simulink model "SVM"  (R2018b)
settings: Solver=VariableStepAuto  StartTime=0.0  StopTime=0.1  FixedStep=1/100000000  RelTol=1e-3
PostLoadFcn:
  | , if any(exist('dsrtsu_mdlpostloadfcn', 'file') ~= 0), dsrtsu_mdlpostloadfcn('Execute', bdroot); end,
values from neighbouring files (symbols this model uses):
  omega = 75    [param.m]
  Vo = 200    [param.m]
libraries: xbsIndex_r4 x2079, xrbsSSR_Library x20, xrbsMath_r4 x11, rtiproclib x6, rtifpgainterfacelib x1, powerlib_meascontrol x1
(part 5 of 23)

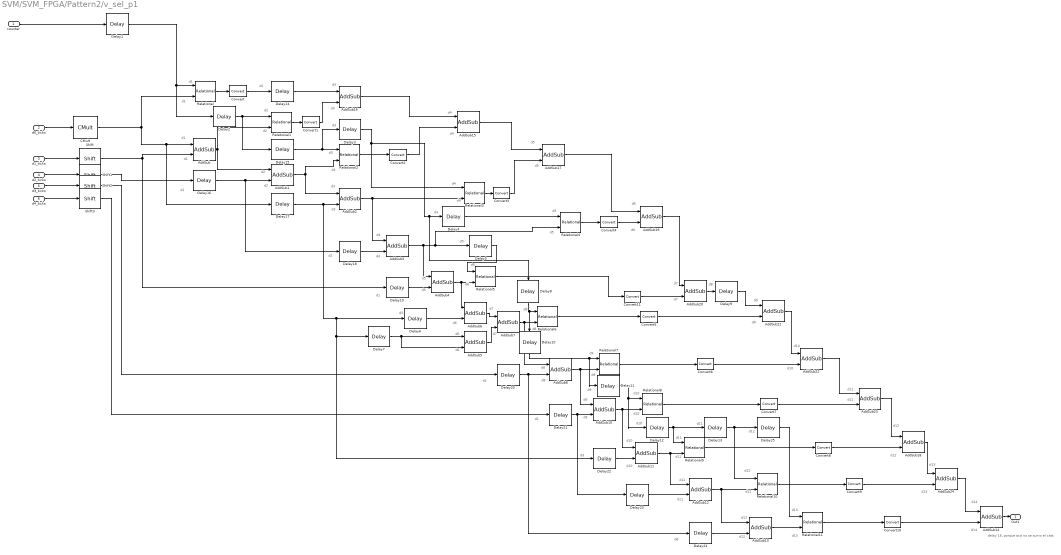
== system SVM/SVM_FPGA/Pattern2/v_sel_p1 ==
  note: d14
  note: d13
  note: d14
  note: d13
  note: d12
  note: d13
  note: d12
  note: d12
  note: d11
  note: d12
  note: d11
  note: d12
  note: d11
  note: d13
  note: d12
  note: d11
  note: d10
  note: d11
  note: d10
  note: d10
  note: d3
  note: d9
  note: d1
  note: d12
  note: d11
  note: d9
  note: d10
  note: d10
  note: d9
  note: d8
  note: d11
  note: d10
  note: d9
  note: d9
  note: d8
  note: d1
  note: d8
  note: d10
  note: d9
  note: d8
  note: d9
  note: d8
  note: d6
  note: d5
  note: d4
  note: d8
  note: d7
  note: d7
  note: d6
  note: d6
  note: d1
  note: d2
  note: d3
  note: d6
  note: d7
  note: d7
  note: d5
  note: d6
  note: d6
  note: d5
  note: d5
  note: d5
  note: d4
  note: d4
  note: d6
  note: d5
  note: d3
  note: d4
  note: d4
  note: d3
  note: d3
  note: d4
  note: d3
  note: d2
  note: d2
  note: d3
  note: d3
  note: d2
  note: d2
  note: d1
  note: d1
  note: d1
  note: d1
  note: d5
  note: d4
  note: d3
  note: d2
  note: d1
  note: delay 16, porque acá no se sumo el cast
  counter : Inport
  d0_ticks : Inport  Port=2
  d1_ticks : Inport  Port=3
  d2_ticks : Inport  Port=4
  d3_ticks : Inport  Port=5
  d4_ticks : Inport  Port=6
  AddSub{,1..8,10..13} (13 alike) : xbsIndex_r4/AddSub  mode=Addition  use_carryin=off  use_carryout=off  en=off  latency=1  precision=Full  arith_type=Unsigned  n_bits=16  bin_pt=14  quantization=Truncate  overflow=Wrap  use_behavioral_HDL=off  hw_selection=Fabric  pipelined=off  dbl_ovrd=off  block_type=addsub
  AddSub{14,18,22..24} (5 alike) : xbsIndex_r4/AddSub  mode=Addition  use_carryin=off  use_carryout=off  en=off  latency=1  precision=User Defined  arith_type=Unsigned  n_bits=4  bin_pt=0  quantization=Truncate  overflow=Wrap  use_behavioral_HDL=off  hw_selection=Fabric  pipelined=off  dbl_ovrd=off  block_type=addsub
  AddSub15 : xbsIndex_r4/AddSub  mode=Addition  use_carryin=off  use_carryout=off  en=off  latency=1  precision=User Defined  arith_type=Unsigned  n_bits=2  bin_pt=0  quantization=Truncate  overflow=Wrap  use_behavioral_HDL=off  hw_selection=Fabric  pipelined=off  dbl_ovrd=off  block_type=addsub
  AddSub16 : xbsIndex_r4/AddSub  mode=Addition  use_carryin=off  use_carryout=off  en=off  latency=1  precision=User Defined  arith_type=Unsigned  n_bits=2  bin_pt=0  quantization=Truncate  overflow=Wrap  use_behavioral_HDL=off  hw_selection=Fabric  pipelined=off  dbl_ovrd=off  block_type=addsub
  AddSub{17,19..21} (4 alike) : xbsIndex_r4/AddSub  mode=Addition  use_carryin=off  use_carryout=off  en=off  latency=1  precision=User Defined  arith_type=Unsigned  n_bits=3  bin_pt=0  quantization=Truncate  overflow=Wrap  use_behavioral_HDL=off  hw_selection=Fabric  pipelined=off  dbl_ovrd=off  block_type=addsub
  CMult : xbsIndex_r4/CMult  const=1/6  gui_display_data_type=Fixed-point  const_n_bits=16  const_bin_pt=16  float_type=Single  exp_bits=8  fraction_bits=24  en=off  latency=1  precision=Full  arith_type="Signed  (2's comp)"  n_bits=16  bin_pt=14  quantization=Truncate  overflow=Wrap  use_behavioral_HDL=off  mem_type=Distributed RAM  pipeline=off  dbl_ovrd=off  block_type=cmult
  Convert{,1..11} (12 alike) : xbsIndex_r4/Convert  gui_display_data_type=Fixed-point  arith_type="Signed  (2's comp)"  n_bits=1  bin_pt=0  float_type=Single  exp_bits=8  fraction_bits=24  quantization=Truncate  overflow=Wrap  en=off  latency=1  pipeline=off  dbl_ovrd=off  block_type=convert
  Delay{1..5,9..16,25} (14 alike) : xbsIndex_r4/Delay  rst=off  infoeditControl=Selection of Reset will increase slice count due to use of real FFs and instead of SRLs  en=off  latency=1  reg_retiming=off  dbl_ovrd=off  block_type=delay
  Delay17 : xbsIndex_r4/Delay  rst=off  infoeditControl=Selection of Reset will increase slice count due to use of real FFs and instead of SRLs  en=off  latency=2  reg_retiming=off  dbl_ovrd=off  block_type=delay
  Delay18 : xbsIndex_r4/Delay  rst=off  infoeditControl=Selection of Reset will increase slice count due to use of real FFs and instead of SRLs  en=off  latency=2  reg_retiming=off  dbl_ovrd=off  block_type=delay
  Delay19 : xbsIndex_r4/Delay  rst=off  infoeditControl=Selection of Reset will increase slice count due to use of real FFs and instead of SRLs  en=off  latency=4  reg_retiming=off  dbl_ovrd=off  block_type=delay
  Delay20 : xbsIndex_r4/Delay  rst=off  infoeditControl=Selection of Reset will increase slice count due to use of real FFs and instead of SRLs  en=off  latency=7  reg_retiming=off  dbl_ovrd=off  block_type=delay
  Delay21 : xbsIndex_r4/Delay  rst=off  infoeditControl=Selection of Reset will increase slice count due to use of real FFs and instead of SRLs  en=off  latency=8  reg_retiming=off  dbl_ovrd=off  block_type=delay
  Delay22 : xbsIndex_r4/Delay  rst=off  infoeditControl=Selection of Reset will increase slice count due to use of real FFs and instead of SRLs  en=off  latency=7  reg_retiming=off  dbl_ovrd=off  block_type=delay
  Delay23 : xbsIndex_r4/Delay  rst=off  infoeditControl=Selection of Reset will increase slice count due to use of real FFs and instead of SRLs  en=off  latency=2  reg_retiming=off  dbl_ovrd=off  block_type=delay
  Delay24 : xbsIndex_r4/Delay  rst=off  infoeditControl=Selection of Reset will increase slice count due to use of real FFs and instead of SRLs  en=off  latency=4  reg_retiming=off  dbl_ovrd=off  block_type=delay
  Delay6 : xbsIndex_r4/Delay  rst=off  infoeditControl=Selection of Reset will increase slice count due to use of real FFs and instead of SRLs  en=off  latency=3  reg_retiming=off  dbl_ovrd=off  block_type=delay
  Delay7 : xbsIndex_r4/Delay  rst=off  infoeditControl=Selection of Reset will increase slice count due to use of real FFs and instead of SRLs  en=off  latency=3  reg_retiming=off  dbl_ovrd=off  block_type=delay
  Delay8 : xbsIndex_r4/Delay  rst=off  infoeditControl=Selection of Reset will increase slice count due to use of real FFs and instead of SRLs  en=off  latency=4  reg_retiming=off  dbl_ovrd=off  block_type=delay
  Relational{,1..11} (12 alike) : xbsIndex_r4/Relational  mode=a>b  op_type=Bool  en=off  latency=1  dbl_ovrd=off  block_type=relational
  Shift{,1..3} (4 alike) : xbsIndex_r4/Shift  shift_dir=Right  shift_bits=1  en=off  latency=1  precision=Full  arith_type="Signed  (2's comp)"  n_bits=16  bin_pt=14  quantization=Truncate  overflow=Wrap  dbl_ovrd=off  block_type=shift
  Out1 : Outport
  wires:
  AddSub15/1 -> AddSub17/1
  AddSub16/1 -> AddSub15/1
  AddSub24/1 -> AddSub14/1
  Shift1/1 -> Delay16/1
  Delay17/1 -> AddSub2/2, Delay22/1, Delay7/1, Delay6/1
  AddSub20/1 -> Delay9/1
  AddSub11/1 -> AddSub12/1, Relational9/2
  AddSub6/1 -> AddSub7/1
  Relational4/1 -> Convert4/1
  Delay19/1 -> AddSub4/2
  counter/1 -> Delay1/1
  AddSub18/1 -> AddSub24/1
  CMult/1 -> Delay17/1, AddSub/1, Relational/2
  Shift/1 -> Delay19/1, AddSub/2
  Delay20/1 -> Delay24/1, AddSub8/2
  Delay22/1 -> AddSub11/2
  AddSub5/1 -> AddSub7/2
  Delay16/1 -> Delay18/1, AddSub1/2
  Relational1/1 -> Convert1/1
  AddSub12/1 -> AddSub13/1, Relational10/2
  Relational8/1 -> Convert7/1
  AddSub23/1 -> AddSub18/1
  Delay23/1 -> AddSub12/2
  Relational5/1 -> Convert11/1
  AddSub4/1 -> AddSub6/1, Relational5/2
  AddSub/1 -> AddSub1/1, Relational1/2
  AddSub8/1 -> AddSub10/1, Relational7/2
  Delay15/1 -> Delay3/1, Relational2/1
  AddSub7/1 -> Relational6/2, AddSub8/1
  Relational2/1 -> Convert2/1
  Delay21/1 -> Delay23/1, AddSub10/2
  d3_ticks/1 -> Shift2/1
  Relational6/1 -> Convert5/1
  Relational10/1 -> Convert9/1
  AddSub19/1 -> AddSub20/1
  Delay18/1 -> AddSub3/2
  AddSub17/1 -> AddSub19/1
  Relational/1 -> Convert/1
  AddSub1/1 -> AddSub2/1, Relational2/2
  AddSub22/1 -> AddSub23/1
  AddSub3/1 -> AddSub4/1, Relational4/2, Delay5/1
  AddSub10/1 -> AddSub11/1, Relational8/2
  d1_ticks/1 -> Shift/1
  AddSub13/1 -> Relational11/2
  Delay24/1 -> AddSub13/2
  d0_ticks/1 -> CMult/1
  Shift2/1 -> Delay20/1
  Relational3/1 -> Convert3/1
  Relational11/1 -> Convert10/1
  AddSub2/1 -> AddSub3/1, Relational3/2
  AddSub21/1 -> AddSub22/1
  Shift3/1 -> Delay21/1
  Relational7/1 -> Convert6/1
  Relational9/1 -> Convert8/1
  AddSub14/1 -> Out1/1
  d4_ticks/1 -> Shift3/1
  d2_ticks/1 -> Shift1/1
  Delay1/1 -> Delay2/1, Relational/1
  Delay2/1 -> Relational1/1, Delay15/1
  Delay3/1 -> Relational3/1, Delay8/1, Delay4/1
  Delay4/1 -> Relational4/1
  Delay5/1 -> Relational5/1
  Delay6/1 -> AddSub6/2
  Delay7/1 -> AddSub5/2, AddSub5/1
  Delay8/1 -> Delay10/1, Relational6/1
  Delay9/1 -> AddSub21/1
  Delay10/1 -> Delay11/1, Relational7/1
  Delay11/1 -> Delay12/1, Relational8/1
  Delay12/1 -> Relational9/1, Delay13/1
  Delay13/1 -> Relational10/1, Delay25/1
  Delay25/1 -> Relational11/1
  Delay14/1 -> AddSub16/1
  Convert1/1 -> AddSub16/2
  Convert2/1 -> AddSub15/2
  Convert3/1 -> AddSub17/2
  Convert4/1 -> AddSub19/2
  Convert5/1 -> AddSub21/2
  Convert6/1 -> AddSub22/2
  Convert7/1 -> AddSub23/2
  Convert8/1 -> AddSub18/2
  Convert9/1 -> AddSub24/2
  Convert10/1 -> AddSub14/2
  Convert11/1 -> AddSub20/2
  Convert/1 -> Delay14/1

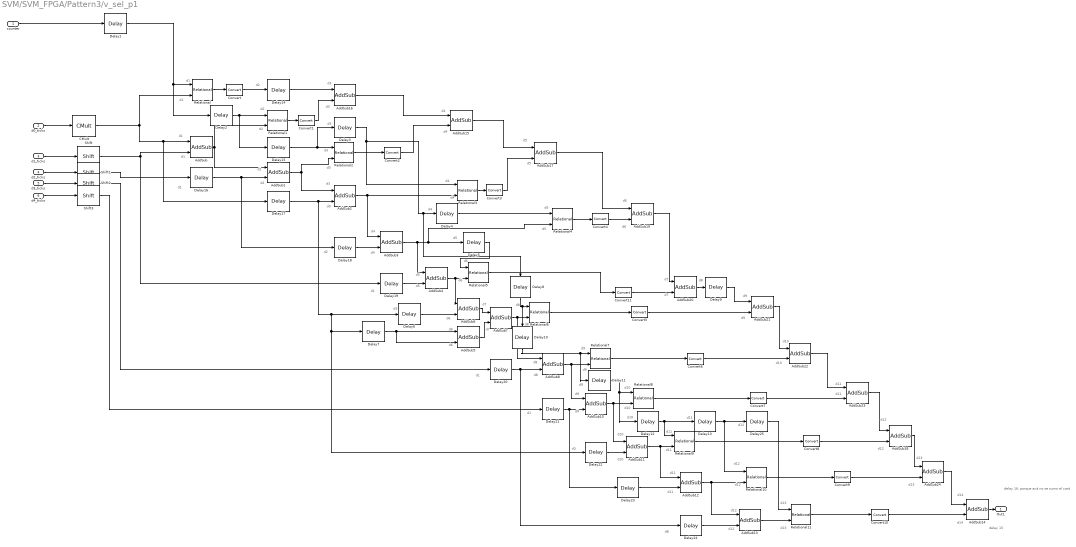
== system SVM/SVM_FPGA/Pattern3/v_sel_p1 ==
  note: delay 15
  note: d1
  note: d2
  note: d3
  note: d4
  note: d5
  note: d1
  note: d1
  note: d1
  note: d1
  note: d2
  note: d2
  note: d3
  note: d3
  note: d2
  note: d2
  note: d3
  note: d4
  note: d3
  note: d3
  note: d4
  note: d4
  note: d3
  note: d5
  note: d6
  note: d4
  note: d4
  note: d5
  note: d5
  note: d5
  note: d6
  note: d6
  note: d5
  note: d7
  note: d7
  note: d6
  note: d3
  note: d2
  note: d1
  note: d6
  note: d6
  note: d7
  note: d7
  note: d8
  note: d4
  note: d5
  note: d6
  note: d8
  note: d9
  note: d8
  note: d9
  note: d10
  note: d8
  note: d1
  note: d8
  note: d9
  note: d9
  note: d10
  note: d11
  note: d8
  note: d9
  note: d10
  note: d10
  note: d9
  note: d11
  note: d12
  note: d1
  note: d9
  note: d3
  note: d10
  note: d10
  note: d11
  note: d10
  note: d11
  note: d12
  note: d13
  note: d11
  note: d12
  note: d11
  note: d12
  note: d11
  note: d12
  note: d12
  note: d13
  note: d12
  note: d13
  note: d14
  note: d13
  note: d14
  note: delay 16, porque acá no se sumo el cast
  counter : Inport
  d0_ticks : Inport  Port=2
  d1_ticks : Inport  Port=3
  d2_ticks : Inport  Port=4
  d3_ticks : Inport  Port=5
  d4_ticks : Inport  Port=6
  AddSub{,1..8,10..13} (13 alike) : xbsIndex_r4/AddSub  mode=Addition  use_carryin=off  use_carryout=off  en=off  latency=1  precision=Full  arith_type=Unsigned  n_bits=16  bin_pt=14  quantization=Truncate  overflow=Wrap  use_behavioral_HDL=off  hw_selection=Fabric  pipelined=off  dbl_ovrd=off  block_type=addsub
  AddSub{14,18,22..24} (5 alike) : xbsIndex_r4/AddSub  mode=Addition  use_carryin=off  use_carryout=off  en=off  latency=1  precision=User Defined  arith_type=Unsigned  n_bits=4  bin_pt=0  quantization=Truncate  overflow=Wrap  use_behavioral_HDL=off  hw_selection=Fabric  pipelined=off  dbl_ovrd=off  block_type=addsub
  AddSub15 : xbsIndex_r4/AddSub  mode=Addition  use_carryin=off  use_carryout=off  en=off  latency=1  precision=User Defined  arith_type=Unsigned  n_bits=2  bin_pt=0  quantization=Truncate  overflow=Wrap  use_behavioral_HDL=off  hw_selection=Fabric  pipelined=off  dbl_ovrd=off  block_type=addsub
  AddSub16 : xbsIndex_r4/AddSub  mode=Addition  use_carryin=off  use_carryout=off  en=off  latency=1  precision=User Defined  arith_type=Unsigned  n_bits=2  bin_pt=0  quantization=Truncate  overflow=Wrap  use_behavioral_HDL=off  hw_selection=Fabric  pipelined=off  dbl_ovrd=off  block_type=addsub
  AddSub{17,19..21} (4 alike) : xbsIndex_r4/AddSub  mode=Addition  use_carryin=off  use_carryout=off  en=off  latency=1  precision=User Defined  arith_type=Unsigned  n_bits=3  bin_pt=0  quantization=Truncate  overflow=Wrap  use_behavioral_HDL=off  hw_selection=Fabric  pipelined=off  dbl_ovrd=off  block_type=addsub
  CMult : xbsIndex_r4/CMult  const=1/6  gui_display_data_type=Fixed-point  const_n_bits=16  const_bin_pt=16  float_type=Single  exp_bits=8  fraction_bits=24  en=off  latency=1  precision=Full  arith_type="Signed  (2's comp)"  n_bits=16  bin_pt=14  quantization=Truncate  overflow=Wrap  use_behavioral_HDL=off  mem_type=Distributed RAM  pipeline=off  dbl_ovrd=off  block_type=cmult
  Convert{,1..11} (12 alike) : xbsIndex_r4/Convert  gui_display_data_type=Fixed-point  arith_type="Signed  (2's comp)"  n_bits=1  bin_pt=0  float_type=Single  exp_bits=8  fraction_bits=24  quantization=Truncate  overflow=Wrap  en=off  latency=1  pipeline=off  dbl_ovrd=off  block_type=convert
  Delay{1..5,9..16,25} (14 alike) : xbsIndex_r4/Delay  rst=off  infoeditControl=Selection of Reset will increase slice count due to use of real FFs and instead of SRLs  en=off  latency=1  reg_retiming=off  dbl_ovrd=off  block_type=delay
  Delay17 : xbsIndex_r4/Delay  rst=off  infoeditControl=Selection of Reset will increase slice count due to use of real FFs and instead of SRLs  en=off  latency=2  reg_retiming=off  dbl_ovrd=off  block_type=delay
  Delay18 : xbsIndex_r4/Delay  rst=off  infoeditControl=Selection of Reset will increase slice count due to use of real FFs and instead of SRLs  en=off  latency=2  reg_retiming=off  dbl_ovrd=off  block_type=delay
  Delay19 : xbsIndex_r4/Delay  rst=off  infoeditControl=Selection of Reset will increase slice count due to use of real FFs and instead of SRLs  en=off  latency=4  reg_retiming=off  dbl_ovrd=off  block_type=delay
  Delay20 : xbsIndex_r4/Delay  rst=off  infoeditControl=Selection of Reset will increase slice count due to use of real FFs and instead of SRLs  en=off  latency=7  reg_retiming=off  dbl_ovrd=off  block_type=delay
  Delay21 : xbsIndex_r4/Delay  rst=off  infoeditControl=Selection of Reset will increase slice count due to use of real FFs and instead of SRLs  en=off  latency=8  reg_retiming=off  dbl_ovrd=off  block_type=delay
  Delay22 : xbsIndex_r4/Delay  rst=off  infoeditControl=Selection of Reset will increase slice count due to use of real FFs and instead of SRLs  en=off  latency=7  reg_retiming=off  dbl_ovrd=off  block_type=delay
  Delay23 : xbsIndex_r4/Delay  rst=off  infoeditControl=Selection of Reset will increase slice count due to use of real FFs and instead of SRLs  en=off  latency=2  reg_retiming=off  dbl_ovrd=off  block_type=delay
  Delay24 : xbsIndex_r4/Delay  rst=off  infoeditControl=Selection of Reset will increase slice count due to use of real FFs and instead of SRLs  en=off  latency=4  reg_retiming=off  dbl_ovrd=off  block_type=delay
  Delay6 : xbsIndex_r4/Delay  rst=off  infoeditControl=Selection of Reset will increase slice count due to use of real FFs and instead of SRLs  en=off  latency=3  reg_retiming=off  dbl_ovrd=off  block_type=delay
  Delay7 : xbsIndex_r4/Delay  rst=off  infoeditControl=Selection of Reset will increase slice count due to use of real FFs and instead of SRLs  en=off  latency=3  reg_retiming=off  dbl_ovrd=off  block_type=delay
  Delay8 : xbsIndex_r4/Delay  rst=off  infoeditControl=Selection of Reset will increase slice count due to use of real FFs and instead of SRLs  en=off  latency=4  reg_retiming=off  dbl_ovrd=off  block_type=delay
  Relational{,1..11} (12 alike) : xbsIndex_r4/Relational  mode=a>b  op_type=Bool  en=off  latency=1  dbl_ovrd=off  block_type=relational
  Shift{,1..3} (4 alike) : xbsIndex_r4/Shift  shift_dir=Right  shift_bits=1  en=off  latency=1  precision=Full  arith_type="Signed  (2's comp)"  n_bits=16  bin_pt=14  quantization=Truncate  overflow=Wrap  dbl_ovrd=off  block_type=shift
  Out1 : Outport
  wires:
  Convert/1 -> Delay14/1
  Convert11/1 -> AddSub20/2
  Convert10/1 -> AddSub14/2
  Convert9/1 -> AddSub24/2
  Convert8/1 -> AddSub18/2
  Convert7/1 -> AddSub23/2
  Convert6/1 -> AddSub22/2
  Convert5/1 -> AddSub21/2
  Convert4/1 -> AddSub19/2
  Convert3/1 -> AddSub17/2
  Convert2/1 -> AddSub15/2
  Convert1/1 -> AddSub16/2
  Delay14/1 -> AddSub16/1
  Delay25/1 -> Relational11/1
  Delay13/1 -> Delay25/1, Relational10/1
  Delay12/1 -> Delay13/1, Relational9/1
  Delay11/1 -> Relational8/1, Delay12/1
  Delay10/1 -> Relational7/1, Delay11/1
  Delay9/1 -> AddSub21/1
  Delay8/1 -> Relational6/1, Delay10/1
  Delay7/1 -> AddSub5/1, AddSub5/2
  Delay6/1 -> AddSub6/2
  Delay5/1 -> Relational5/1
  Delay4/1 -> Relational4/1
  Delay3/1 -> Delay4/1, Delay8/1, Relational3/1
  Delay2/1 -> Delay15/1, Relational1/1
  Delay1/1 -> Relational/1, Delay2/1
  d2_ticks/1 -> Shift1/1
  d4_ticks/1 -> Shift3/1
  AddSub14/1 -> Out1/1
  Relational9/1 -> Convert8/1
  Relational7/1 -> Convert6/1
  Shift3/1 -> Delay21/1
  AddSub21/1 -> AddSub22/1
  AddSub2/1 -> Relational3/2, AddSub3/1
  Relational11/1 -> Convert10/1
  Relational3/1 -> Convert3/1
  Shift2/1 -> Delay20/1
  d0_ticks/1 -> CMult/1
  Delay24/1 -> AddSub13/2
  AddSub13/1 -> Relational11/2
  d1_ticks/1 -> Shift/1
  AddSub10/1 -> Relational8/2, AddSub11/1
  AddSub3/1 -> Delay5/1, Relational4/2, AddSub4/1
  AddSub22/1 -> AddSub23/1
  AddSub1/1 -> Relational2/2, AddSub2/1
  Relational/1 -> Convert/1
  AddSub17/1 -> AddSub19/1
  Delay18/1 -> AddSub3/2
  AddSub19/1 -> AddSub20/1
  Relational10/1 -> Convert9/1
  Relational6/1 -> Convert5/1
  d3_ticks/1 -> Shift2/1
  Delay21/1 -> AddSub10/2, Delay23/1
  Relational2/1 -> Convert2/1
  AddSub7/1 -> AddSub8/1, Relational6/2
  Delay15/1 -> Relational2/1, Delay3/1
  AddSub8/1 -> Relational7/2, AddSub10/1
  AddSub/1 -> Relational1/2, AddSub1/1
  AddSub4/1 -> Relational5/2, AddSub6/1
  Relational5/1 -> Convert11/1
  Delay23/1 -> AddSub12/2
  AddSub23/1 -> AddSub18/1
  Relational8/1 -> Convert7/1
  AddSub12/1 -> Relational10/2, AddSub13/1
  Relational1/1 -> Convert1/1
  Delay16/1 -> AddSub1/2, Delay18/1
  AddSub5/1 -> AddSub7/2
  Delay22/1 -> AddSub11/2
  Delay20/1 -> AddSub8/2, Delay24/1
  Shift/1 -> AddSub/2, Delay19/1
  CMult/1 -> Relational/2, AddSub/1, Delay17/1
  AddSub18/1 -> AddSub24/1
  counter/1 -> Delay1/1
  Delay19/1 -> AddSub4/2
  Relational4/1 -> Convert4/1
  AddSub6/1 -> AddSub7/1
  AddSub11/1 -> Relational9/2, AddSub12/1
  AddSub20/1 -> Delay9/1
  Delay17/1 -> Delay6/1, Delay7/1, Delay22/1, AddSub2/2
  Shift1/1 -> Delay16/1
  AddSub24/1 -> AddSub14/1
  AddSub16/1 -> AddSub15/1
  AddSub15/1 -> AddSub17/1

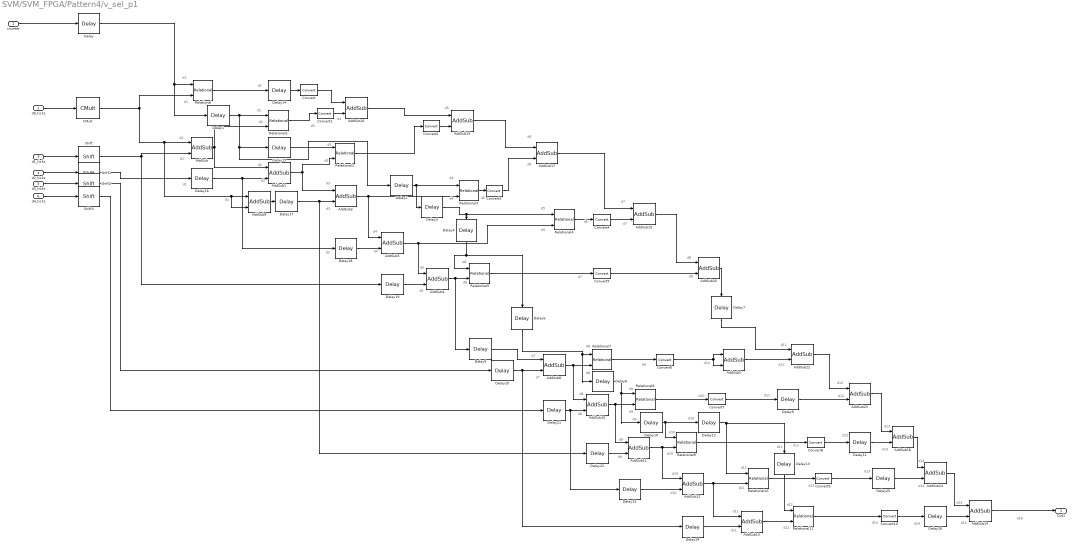
== system SVM/SVM_FPGA/Pattern4/v_sel_p1 ==
  note: d16
  note: d15
  note: d14
  note: d15
  note: d14
  note: d13
  note: d12
  note: d13
  note: d12
  note: d11
  note: d12
  note: d11
  note: d11
  note: d11
  note: d10
  note: d9
  note: d11
  note: d10
  note: d10
  note: d14
  note: d12
  note: d13
  note: d11
  note: d10
  note: d10
  note: d9
  note: d9
  note: d13
  note: d12
  note: d11
  note: d12
  note: d10
  note: d9
  note: d9
  note: d8
  note: d8
  note: d8
  note: d8
  note: d9
  note: d10
  note: d11
  note: d7
  note: d7
  note: d11
  note: d8
  note: d7
  note: d6
  note: d6
  note: d5
  note: d5
  note: d8
  note: d7
  note: d6
  note: d5
  note: d5
  note: d4
  note: d4
  note: d6
  note: d5
  note: d4
  note: d3
  note: d3
  note: d4
  note: d3
  note: d2
  note: d2
  note: d3
  note: d2
  note: d2
  note: d3
  note: d4
  note: d2
  note: d1
  note: d1
  note: d1
  note: d1
  note: d2
  note: d1
  note: d1
  note: d7
  note: d6
  note: d5
  counter : Inport
  d0_ticks : Inport  Port=2
  d1_ticks : Inport  Port=3
  d2_ticks : Inport  Port=4
  d3_ticks : Inport  Port=5
  d4_ticks : Inport  Port=6
  AddSub{,1..5,8..13,16} (13 alike) : xbsIndex_r4/AddSub  mode=Addition  use_carryin=off  use_carryout=off  en=off  latency=1  precision=Full  arith_type=Unsigned  n_bits=16  bin_pt=14  quantization=Truncate  overflow=Wrap  use_behavioral_HDL=off  hw_selection=Fabric  pipelined=off  dbl_ovrd=off  block_type=addsub
  AddSub{14,18,23..24} (4 alike) : xbsIndex_r4/AddSub  mode=Addition  use_carryin=off  use_carryout=off  en=off  latency=1  precision=User Defined  arith_type=Unsigned  n_bits=4  bin_pt=0  quantization=Truncate  overflow=Wrap  use_behavioral_HDL=off  hw_selection=Fabric  pipelined=off  dbl_ovrd=off  block_type=addsub
  AddSub15 : xbsIndex_r4/AddSub  mode=Addition  use_carryin=off  use_carryout=off  en=off  latency=1  precision=User Defined  arith_type=Unsigned  n_bits=2  bin_pt=0  quantization=Truncate  overflow=Wrap  use_behavioral_HDL=off  hw_selection=Fabric  pipelined=off  dbl_ovrd=off  block_type=addsub
  AddSub17 : xbsIndex_r4/AddSub  mode=Addition  use_carryin=off  use_carryout=off  en=off  latency=1  precision=User Defined  arith_type=Unsigned  n_bits=3  bin_pt=0  quantization=Truncate  overflow=Wrap  use_behavioral_HDL=off  hw_selection=Fabric  pipelined=off  dbl_ovrd=off  block_type=addsub
  AddSub19 : xbsIndex_r4/AddSub  mode=Addition  use_carryin=off  use_carryout=off  en=off  latency=1  precision=User Defined  arith_type=Unsigned  n_bits=3  bin_pt=0  quantization=Truncate  overflow=Wrap  use_behavioral_HDL=off  hw_selection=Fabric  pipelined=off  dbl_ovrd=off  block_type=addsub
  AddSub20 : xbsIndex_r4/AddSub  mode=Addition  use_carryin=off  use_carryout=off  en=off  latency=1  precision=User Defined  arith_type=Unsigned  n_bits=5  bin_pt=0  quantization=Truncate  overflow=Wrap  use_behavioral_HDL=off  hw_selection=Fabric  pipelined=off  dbl_ovrd=off  block_type=addsub
  AddSub22 : xbsIndex_r4/AddSub  mode=Addition  use_carryin=off  use_carryout=off  en=off  latency=1  precision=User Defined  arith_type=Unsigned  n_bits=3  bin_pt=0  quantization=Truncate  overflow=Wrap  use_behavioral_HDL=off  hw_selection=Fabric  pipelined=off  dbl_ovrd=off  block_type=addsub
  CMult : xbsIndex_r4/CMult  const=1/6  gui_display_data_type=Fixed-point  const_n_bits=16  const_bin_pt=16  float_type=Single  exp_bits=8  fraction_bits=24  en=off  latency=1  precision=Full  arith_type="Signed  (2's comp)"  n_bits=16  bin_pt=14  quantization=Truncate  overflow=Wrap  use_behavioral_HDL=off  mem_type=Distributed RAM  pipeline=off  dbl_ovrd=off  block_type=cmult
  Convert{,1..10} (11 alike) : xbsIndex_r4/Convert  gui_display_data_type=Fixed-point  arith_type="Signed  (2's comp)"  n_bits=1  bin_pt=0  float_type=Single  exp_bits=8  fraction_bits=24  quantization=Truncate  overflow=Wrap  en=off  latency=1  pipeline=off  dbl_ovrd=off  block_type=convert
  Delay{,1,3..5,8..17,25..26} (17 alike) : xbsIndex_r4/Delay  rst=off  infoeditControl=Selection of Reset will increase slice count due to use of real FFs and instead of SRLs  en=off  latency=1  reg_retiming=off  dbl_ovrd=off  block_type=delay
  Delay{2,6..7,18,23} (5 alike) : xbsIndex_r4/Delay  rst=off  infoeditControl=Selection of Reset will increase slice count due to use of real FFs and instead of SRLs  en=off  latency=2  reg_retiming=off  dbl_ovrd=off  block_type=delay
  Delay19 : xbsIndex_r4/Delay  rst=off  infoeditControl=Selection of Reset will increase slice count due to use of real FFs and instead of SRLs  en=off  latency=4  reg_retiming=off  dbl_ovrd=off  block_type=delay
  Delay20 : xbsIndex_r4/Delay  rst=off  infoeditControl=Selection of Reset will increase slice count due to use of real FFs and instead of SRLs  en=off  latency=6  reg_retiming=off  dbl_ovrd=off  block_type=delay
  Delay21 : xbsIndex_r4/Delay  rst=off  infoeditControl=Selection of Reset will increase slice count due to use of real FFs and instead of SRLs  en=off  latency=7  reg_retiming=off  dbl_ovrd=off  block_type=delay
  Delay22 : xbsIndex_r4/Delay  rst=off  infoeditControl=Selection of Reset will increase slice count due to use of real FFs and instead of SRLs  en=off  latency=6  reg_retiming=off  dbl_ovrd=off  block_type=delay
  Delay24 : xbsIndex_r4/Delay  rst=off  infoeditControl=Selection of Reset will increase slice count due to use of real FFs and instead of SRLs  en=off  latency=4  reg_retiming=off  dbl_ovrd=off  block_type=delay
  Relational{,1..5,7..11} (11 alike) : xbsIndex_r4/Relational  mode=a>b  op_type=Bool  en=off  latency=1  dbl_ovrd=off  block_type=relational
  Shift{,1..3} (4 alike) : xbsIndex_r4/Shift  shift_dir=Right  shift_bits=1  en=off  latency=1  precision=Full  arith_type="Signed  (2's comp)"  n_bits=16  bin_pt=14  quantization=Truncate  overflow=Wrap  dbl_ovrd=off  block_type=shift
  Out1 : Outport
  wires:
  AddSub15/1 -> AddSub17/1
  AddSub24/1 -> AddSub14/1
  Shift1/1 -> Delay16/1
  Delay17/1 -> AddSub2/2, Delay22/1
  AddSub11/1 -> AddSub12/1, Relational9/2
  Relational4/1 -> Convert4/1
  Delay19/1 -> AddSub4/2
  counter/1 -> Delay/1
  AddSub18/1 -> AddSub24/1
  CMult/1 -> Relational/2, AddSub9/2, AddSub9/1, AddSub/1
  Shift/1 -> Delay19/1, AddSub/2
  Delay20/1 -> Delay24/1, AddSub8/2
  Delay22/1 -> AddSub11/2
  Delay16/1 -> Delay18/1, AddSub1/2
  Relational1/1 -> Convert1/1
  AddSub12/1 -> AddSub13/1, Relational10/2
  Relational8/1 -> Convert7/1
  AddSub23/1 -> AddSub18/1
  Delay23/1 -> AddSub12/2
  Relational5/1 -> Convert5/1
  AddSub4/1 -> Delay5/1, Relational5/2
  AddSub/1 -> AddSub1/1, Relational1/2
  AddSub8/1 -> AddSub10/1, Relational7/2
  Delay15/1 -> Relational2/1
  Relational2/1 -> Convert2/1
  Delay14/1 -> Convert/1
  Delay21/1 -> Delay23/1, AddSub10/2
  d3_ticks/1 -> Shift2/1
  Relational10/1 -> Convert9/1
  AddSub19/1 -> AddSub20/1
  Delay18/1 -> AddSub3/2
  AddSub17/1 -> AddSub19/1
  Relational/1 -> Delay14/1
  AddSub1/1 -> AddSub2/1, Relational2/2
  AddSub22/1 -> AddSub23/1
  AddSub3/1 -> AddSub4/1, Relational4/2
  AddSub10/1 -> AddSub11/1, Relational8/2
  d1_ticks/1 -> Shift/1
  AddSub13/1 -> Relational11/2
  Delay24/1 -> AddSub13/2
  Shift2/1 -> Delay20/1
  Relational3/1 -> Convert3/1
  Relational11/1 -> Convert10/1
  AddSub2/1 -> AddSub3/1, Relational3/2
  AddSub20/1 -> Delay7/1
  Shift3/1 -> Delay21/1
  Relational7/1 -> Convert6/1
  Relational9/1 -> Convert8/1
  AddSub14/1 -> Out1/1
  d4_ticks/1 -> Shift3/1
  d2_ticks/1 -> Shift1/1
  AddSub9/1 -> Delay17/1
  AddSub5/1 -> AddSub22/2
  d0_ticks/1 -> CMult/1
  Convert/1 -> AddSub16/1
  Convert1/1 -> AddSub16/2
  AddSub16/1 -> AddSub15/1
  Convert2/1 -> AddSub15/2
  Convert3/1 -> AddSub17/2
  Convert4/1 -> AddSub19/2
  Convert5/1 -> AddSub20/2
  Convert6/1 -> AddSub5/1, AddSub5/2
  Convert7/1 -> Delay9/1
  Convert8/1 -> Delay11/1
  Convert9/1 -> Delay25/1
  Convert10/1 -> Delay26/1
  Delay/1 -> Delay1/1, Relational/1
  Delay1/1 -> Relational1/1, Delay15/1, Delay2/1
  Delay2/1 -> Relational3/1, Delay3/1
  Delay3/1 -> Relational4/1, Delay4/1
  Delay4/1 -> Delay6/1, Relational5/1
  Delay5/1 -> AddSub8/1
  Delay6/1 -> Delay8/1, Relational7/1
  Delay7/1 -> AddSub22/1
  Delay8/1 -> Delay10/1, Relational8/1
  Delay9/1 -> AddSub23/2
  Delay10/1 -> Relational9/1, Delay12/1
  Delay11/1 -> AddSub18/2
  Delay12/1 -> Delay13/1, Relational10/1
  Delay13/1 -> Relational11/1
  Delay25/1 -> AddSub24/2
  Delay26/1 -> AddSub14/2

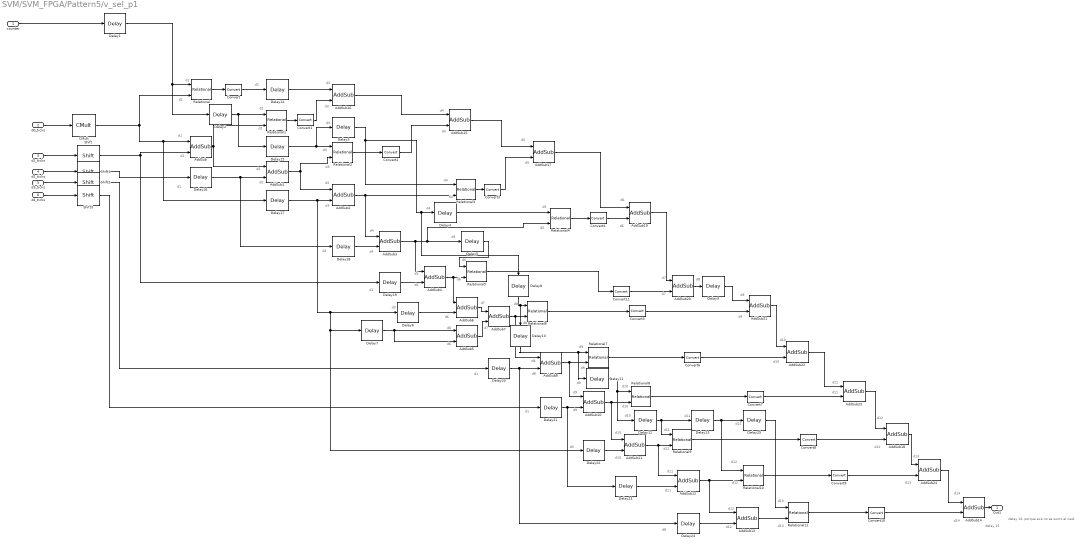
== system SVM/SVM_FPGA/Pattern5/v_sel_p1 ==
  note: d14
  note: d13
  note: d14
  note: d13
  note: d12
  note: d13
  note: d12
  note: d12
  note: d11
  note: d12
  note: d11
  note: d12
  note: d11
  note: d13
  note: d12
  note: d11
  note: d10
  note: d11
  note: d10
  note: d10
  note: d3
  note: d9
  note: d1
  note: d12
  note: d11
  note: d9
  note: d10
  note: d10
  note: d9
  note: d8
  note: d11
  note: d10
  note: d9
  note: d9
  note: d8
  note: d1
  note: d8
  note: d10
  note: d9
  note: d8
  note: d9
  note: d8
  note: d6
  note: d5
  note: d4
  note: d8
  note: d7
  note: d7
  note: d6
  note: d6
  note: d1
  note: d2
  note: d3
  note: d6
  note: d7
  note: d7
  note: d5
  note: d6
  note: d6
  note: d5
  note: d5
  note: d5
  note: d4
  note: d4
  note: d6
  note: d5
  note: d3
  note: d4
  note: d4
  note: d3
  note: d3
  note: d4
  note: d3
  note: d2
  note: d2
  note: d3
  note: d3
  note: d2
  note: d2
  note: d1
  note: d1
  note: d1
  note: d1
  note: d5
  note: d4
  note: d3
  note: d2
  note: d1
  note: delay 15
  note: delay 16, porque acá no se sumo el cast
  counter : Inport
  d0_ticks : Inport  Port=2
  d1_ticks : Inport  Port=3
  d2_ticks : Inport  Port=4
  d3_ticks : Inport  Port=5
  d4_ticks : Inport  Port=6
  AddSub{,1..8,10..13} (13 alike) : xbsIndex_r4/AddSub  mode=Addition  use_carryin=off  use_carryout=off  en=off  latency=1  precision=Full  arith_type=Unsigned  n_bits=16  bin_pt=14  quantization=Truncate  overflow=Wrap  use_behavioral_HDL=off  hw_selection=Fabric  pipelined=off  dbl_ovrd=off  block_type=addsub
  AddSub{14,18,22..24} (5 alike) : xbsIndex_r4/AddSub  mode=Addition  use_carryin=off  use_carryout=off  en=off  latency=1  precision=User Defined  arith_type=Unsigned  n_bits=4  bin_pt=0  quantization=Truncate  overflow=Wrap  use_behavioral_HDL=off  hw_selection=Fabric  pipelined=off  dbl_ovrd=off  block_type=addsub
  AddSub15 : xbsIndex_r4/AddSub  mode=Addition  use_carryin=off  use_carryout=off  en=off  latency=1  precision=User Defined  arith_type=Unsigned  n_bits=2  bin_pt=0  quantization=Truncate  overflow=Wrap  use_behavioral_HDL=off  hw_selection=Fabric  pipelined=off  dbl_ovrd=off  block_type=addsub
  AddSub16 : xbsIndex_r4/AddSub  mode=Addition  use_carryin=off  use_carryout=off  en=off  latency=1  precision=User Defined  arith_type=Unsigned  n_bits=2  bin_pt=0  quantization=Truncate  overflow=Wrap  use_behavioral_HDL=off  hw_selection=Fabric  pipelined=off  dbl_ovrd=off  block_type=addsub
  AddSub{17,19..21} (4 alike) : xbsIndex_r4/AddSub  mode=Addition  use_carryin=off  use_carryout=off  en=off  latency=1  precision=User Defined  arith_type=Unsigned  n_bits=3  bin_pt=0  quantization=Truncate  overflow=Wrap  use_behavioral_HDL=off  hw_selection=Fabric  pipelined=off  dbl_ovrd=off  block_type=addsub
  CMult : xbsIndex_r4/CMult  const=1/6  gui_display_data_type=Fixed-point  const_n_bits=16  const_bin_pt=16  float_type=Single  exp_bits=8  fraction_bits=24  en=off  latency=1  precision=Full  arith_type="Signed  (2's comp)"  n_bits=16  bin_pt=14  quantization=Truncate  overflow=Wrap  use_behavioral_HDL=off  mem_type=Distributed RAM  pipeline=off  dbl_ovrd=off  block_type=cmult
  Convert{,1..11} (12 alike) : xbsIndex_r4/Convert  gui_display_data_type=Fixed-point  arith_type="Signed  (2's comp)"  n_bits=1  bin_pt=0  float_type=Single  exp_bits=8  fraction_bits=24  quantization=Truncate  overflow=Wrap  en=off  latency=1  pipeline=off  dbl_ovrd=off  block_type=convert
  Delay{1..5,9..16,25} (14 alike) : xbsIndex_r4/Delay  rst=off  infoeditControl=Selection of Reset will increase slice count due to use of real FFs and instead of SRLs  en=off  latency=1  reg_retiming=off  dbl_ovrd=off  block_type=delay
  Delay17 : xbsIndex_r4/Delay  rst=off  infoeditControl=Selection of Reset will increase slice count due to use of real FFs and instead of SRLs  en=off  latency=2  reg_retiming=off  dbl_ovrd=off  block_type=delay
  Delay18 : xbsIndex_r4/Delay  rst=off  infoeditControl=Selection of Reset will increase slice count due to use of real FFs and instead of SRLs  en=off  latency=2  reg_retiming=off  dbl_ovrd=off  block_type=delay
  Delay19 : xbsIndex_r4/Delay  rst=off  infoeditControl=Selection of Reset will increase slice count due to use of real FFs and instead of SRLs  en=off  latency=4  reg_retiming=off  dbl_ovrd=off  block_type=delay
  Delay20 : xbsIndex_r4/Delay  rst=off  infoeditControl=Selection of Reset will increase slice count due to use of real FFs and instead of SRLs  en=off  latency=7  reg_retiming=off  dbl_ovrd=off  block_type=delay
  Delay21 : xbsIndex_r4/Delay  rst=off  infoeditControl=Selection of Reset will increase slice count due to use of real FFs and instead of SRLs  en=off  latency=8  reg_retiming=off  dbl_ovrd=off  block_type=delay
  Delay22 : xbsIndex_r4/Delay  rst=off  infoeditControl=Selection of Reset will increase slice count due to use of real FFs and instead of SRLs  en=off  latency=7  reg_retiming=off  dbl_ovrd=off  block_type=delay
  Delay23 : xbsIndex_r4/Delay  rst=off  infoeditControl=Selection of Reset will increase slice count due to use of real FFs and instead of SRLs  en=off  latency=2  reg_retiming=off  dbl_ovrd=off  block_type=delay
  Delay24 : xbsIndex_r4/Delay  rst=off  infoeditControl=Selection of Reset will increase slice count due to use of real FFs and instead of SRLs  en=off  latency=4  reg_retiming=off  dbl_ovrd=off  block_type=delay
  Delay6 : xbsIndex_r4/Delay  rst=off  infoeditControl=Selection of Reset will increase slice count due to use of real FFs and instead of SRLs  en=off  latency=3  reg_retiming=off  dbl_ovrd=off  block_type=delay
  Delay7 : xbsIndex_r4/Delay  rst=off  infoeditControl=Selection of Reset will increase slice count due to use of real FFs and instead of SRLs  en=off  latency=3  reg_retiming=off  dbl_ovrd=off  block_type=delay
  Delay8 : xbsIndex_r4/Delay  rst=off  infoeditControl=Selection of Reset will increase slice count due to use of real FFs and instead of SRLs  en=off  latency=4  reg_retiming=off  dbl_ovrd=off  block_type=delay
  Relational{,1..11} (12 alike) : xbsIndex_r4/Relational  mode=a>b  op_type=Bool  en=off  latency=1  dbl_ovrd=off  block_type=relational
  Shift{,1..3} (4 alike) : xbsIndex_r4/Shift  shift_dir=Right  shift_bits=1  en=off  latency=1  precision=Full  arith_type="Signed  (2's comp)"  n_bits=16  bin_pt=14  quantization=Truncate  overflow=Wrap  dbl_ovrd=off  block_type=shift
  Out1 : Outport
  wires:
  AddSub15/1 -> AddSub17/1
  AddSub16/1 -> AddSub15/1
  AddSub24/1 -> AddSub14/1
  Shift1/1 -> Delay16/1
  Delay17/1 -> AddSub2/2, Delay22/1, Delay7/1, Delay6/1
  AddSub20/1 -> Delay9/1
  AddSub11/1 -> AddSub12/1, Relational9/2
  AddSub6/1 -> AddSub7/1
  Relational4/1 -> Convert4/1
  Delay19/1 -> AddSub4/2
  counter/1 -> Delay1/1
  AddSub18/1 -> AddSub24/1
  CMult/1 -> Delay17/1, AddSub/1, Relational/2
  Shift/1 -> Delay19/1, AddSub/2
  Delay20/1 -> Delay24/1, AddSub8/2
  Delay22/1 -> AddSub11/2
  AddSub5/1 -> AddSub7/2
  Delay16/1 -> Delay18/1, AddSub1/2
  Relational1/1 -> Convert1/1
  AddSub12/1 -> AddSub13/1, Relational10/2
  Relational8/1 -> Convert7/1
  AddSub23/1 -> AddSub18/1
  Delay23/1 -> AddSub12/2
  Relational5/1 -> Convert11/1
  AddSub4/1 -> AddSub6/1, Relational5/2
  AddSub/1 -> AddSub1/1, Relational1/2
  AddSub8/1 -> AddSub10/1, Relational7/2
  Delay15/1 -> Delay3/1, Relational2/1
  AddSub7/1 -> Relational6/2, AddSub8/1
  Relational2/1 -> Convert2/1
  Delay21/1 -> Delay23/1, AddSub10/2
  d3_ticks/1 -> Shift2/1
  Relational6/1 -> Convert5/1
  Relational10/1 -> Convert9/1
  AddSub19/1 -> AddSub20/1
  Delay18/1 -> AddSub3/2
  AddSub17/1 -> AddSub19/1
  Relational/1 -> Convert/1
  AddSub1/1 -> AddSub2/1, Relational2/2
  AddSub22/1 -> AddSub23/1
  AddSub3/1 -> AddSub4/1, Relational4/2, Delay5/1
  AddSub10/1 -> AddSub11/1, Relational8/2
  d1_ticks/1 -> Shift/1
  AddSub13/1 -> Relational11/2
  Delay24/1 -> AddSub13/2
  d0_ticks/1 -> CMult/1
  Shift2/1 -> Delay20/1
  Relational3/1 -> Convert3/1
  Relational11/1 -> Convert10/1
  AddSub2/1 -> AddSub3/1, Relational3/2
  AddSub21/1 -> AddSub22/1
  Shift3/1 -> Delay21/1
  Relational7/1 -> Convert6/1
  Relational9/1 -> Convert8/1
  AddSub14/1 -> Out1/1
  d4_ticks/1 -> Shift3/1
  d2_ticks/1 -> Shift1/1
  Delay1/1 -> Delay2/1, Relational/1
  Delay2/1 -> Relational1/1, Delay15/1
  Delay3/1 -> Relational3/1, Delay8/1, Delay4/1
  Delay4/1 -> Relational4/1
  Delay5/1 -> Relational5/1
  Delay6/1 -> AddSub6/2
  Delay7/1 -> AddSub5/2, AddSub5/1
  Delay8/1 -> Delay10/1, Relational6/1
  Delay9/1 -> AddSub21/1
  Delay10/1 -> Delay11/1, Relational7/1
  Delay11/1 -> Delay12/1, Relational8/1
  Delay12/1 -> Relational9/1, Delay13/1
  Delay13/1 -> Relational10/1, Delay25/1
  Delay25/1 -> Relational11/1
  Delay14/1 -> AddSub16/1
  Convert1/1 -> AddSub16/2
  Convert2/1 -> AddSub15/2
  Convert3/1 -> AddSub17/2
  Convert4/1 -> AddSub19/2
  Convert5/1 -> AddSub21/2
  Convert6/1 -> AddSub22/2
  Convert7/1 -> AddSub23/2
  Convert8/1 -> AddSub18/2
  Convert9/1 -> AddSub24/2
  Convert10/1 -> AddSub14/2
  Convert11/1 -> AddSub20/2
  Convert/1 -> Delay14/1

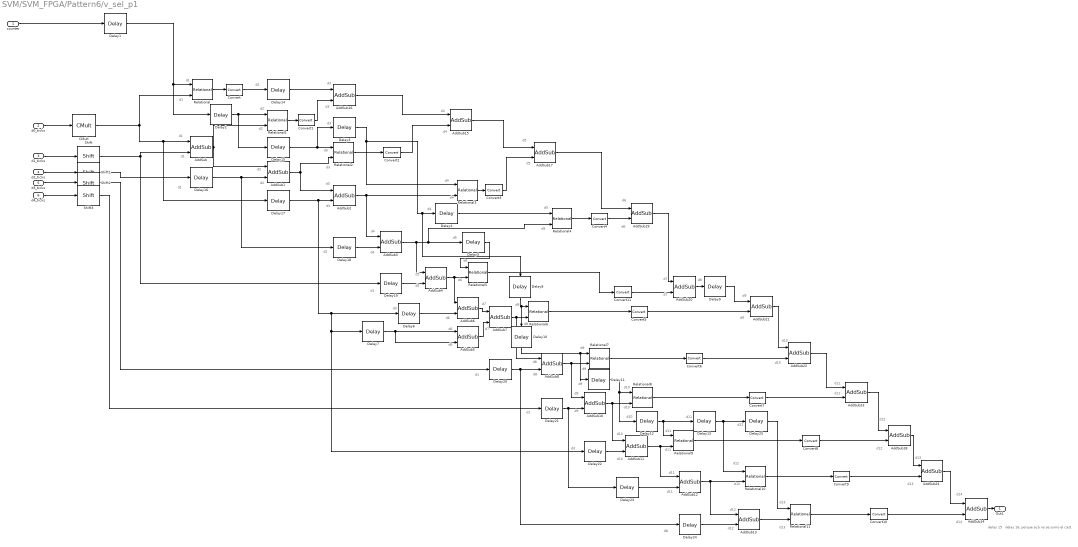
== system SVM/SVM_FPGA/Pattern6/v_sel_p1 ==
  note: delay 15
  note: d1
  note: d2
  note: d3
  note: d4
  note: d5
  note: d1
  note: d1
  note: d1
  note: d1
  note: d2
  note: d2
  note: d3
  note: d3
  note: d2
  note: d2
  note: d3
  note: d4
  note: d3
  note: d3
  note: d4
  note: d4
  note: d3
  note: d5
  note: d6
  note: d4
  note: d4
  note: d5
  note: d5
  note: d5
  note: d6
  note: d6
  note: d5
  note: d7
  note: d7
  note: d6
  note: d3
  note: d2
  note: d1
  note: d6
  note: d6
  note: d7
  note: d7
  note: d8
  note: d4
  note: d5
  note: d6
  note: d8
  note: d9
  note: d8
  note: d9
  note: d10
  note: d8
  note: d1
  note: d8
  note: d9
  note: d9
  note: d10
  note: d11
  note: d8
  note: d9
  note: d10
  note: d10
  note: d9
  note: d11
  note: d12
  note: d1
  note: d9
  note: d3
  note: d10
  note: d10
  note: d11
  note: d10
  note: d11
  note: d12
  note: d13
  note: d11
  note: d12
  note: d11
  note: d12
  note: d11
  note: d12
  note: d12
  note: d13
  note: d12
  note: d13
  note: d14
  note: d13
  note: d14
  note: delay 16, porque acá no se sumo el cast
  counter : Inport
  d0_ticks : Inport  Port=2
  d1_ticks : Inport  Port=3
  d2_ticks : Inport  Port=4
  d3_ticks : Inport  Port=5
  d4_ticks : Inport  Port=6
  AddSub{,1..8,10..13} (13 alike) : xbsIndex_r4/AddSub  mode=Addition  use_carryin=off  use_carryout=off  en=off  latency=1  precision=Full  arith_type=Unsigned  n_bits=16  bin_pt=14  quantization=Truncate  overflow=Wrap  use_behavioral_HDL=off  hw_selection=Fabric  pipelined=off  dbl_ovrd=off  block_type=addsub
  AddSub{14,18,22..24} (5 alike) : xbsIndex_r4/AddSub  mode=Addition  use_carryin=off  use_carryout=off  en=off  latency=1  precision=User Defined  arith_type=Unsigned  n_bits=4  bin_pt=0  quantization=Truncate  overflow=Wrap  use_behavioral_HDL=off  hw_selection=Fabric  pipelined=off  dbl_ovrd=off  block_type=addsub
  AddSub15 : xbsIndex_r4/AddSub  mode=Addition  use_carryin=off  use_carryout=off  en=off  latency=1  precision=User Defined  arith_type=Unsigned  n_bits=2  bin_pt=0  quantization=Truncate  overflow=Wrap  use_behavioral_HDL=off  hw_selection=Fabric  pipelined=off  dbl_ovrd=off  block_type=addsub
  AddSub16 : xbsIndex_r4/AddSub  mode=Addition  use_carryin=off  use_carryout=off  en=off  latency=1  precision=User Defined  arith_type=Unsigned  n_bits=2  bin_pt=0  quantization=Truncate  overflow=Wrap  use_behavioral_HDL=off  hw_selection=Fabric  pipelined=off  dbl_ovrd=off  block_type=addsub
  AddSub{17,19..21} (4 alike) : xbsIndex_r4/AddSub  mode=Addition  use_carryin=off  use_carryout=off  en=off  latency=1  precision=User Defined  arith_type=Unsigned  n_bits=3  bin_pt=0  quantization=Truncate  overflow=Wrap  use_behavioral_HDL=off  hw_selection=Fabric  pipelined=off  dbl_ovrd=off  block_type=addsub
  CMult : xbsIndex_r4/CMult  const=1/6  gui_display_data_type=Fixed-point  const_n_bits=16  const_bin_pt=16  float_type=Single  exp_bits=8  fraction_bits=24  en=off  latency=1  precision=Full  arith_type="Signed  (2's comp)"  n_bits=16  bin_pt=14  quantization=Truncate  overflow=Wrap  use_behavioral_HDL=off  mem_type=Distributed RAM  pipeline=off  dbl_ovrd=off  block_type=cmult
  Convert{,1..11} (12 alike) : xbsIndex_r4/Convert  gui_display_data_type=Fixed-point  arith_type="Signed  (2's comp)"  n_bits=1  bin_pt=0  float_type=Single  exp_bits=8  fraction_bits=24  quantization=Truncate  overflow=Wrap  en=off  latency=1  pipeline=off  dbl_ovrd=off  block_type=convert
  Delay{1..5,9..16,25} (14 alike) : xbsIndex_r4/Delay  rst=off  infoeditControl=Selection of Reset will increase slice count due to use of real FFs and instead of SRLs  en=off  latency=1  reg_retiming=off  dbl_ovrd=off  block_type=delay
  Delay17 : xbsIndex_r4/Delay  rst=off  infoeditControl=Selection of Reset will increase slice count due to use of real FFs and instead of SRLs  en=off  latency=2  reg_retiming=off  dbl_ovrd=off  block_type=delay
  Delay18 : xbsIndex_r4/Delay  rst=off  infoeditControl=Selection of Reset will increase slice count due to use of real FFs and instead of SRLs  en=off  latency=2  reg_retiming=off  dbl_ovrd=off  block_type=delay
  Delay19 : xbsIndex_r4/Delay  rst=off  infoeditControl=Selection of Reset will increase slice count due to use of real FFs and instead of SRLs  en=off  latency=4  reg_retiming=off  dbl_ovrd=off  block_type=delay
  Delay20 : xbsIndex_r4/Delay  rst=off  infoeditControl=Selection of Reset will increase slice count due to use of real FFs and instead of SRLs  en=off  latency=7  reg_retiming=off  dbl_ovrd=off  block_type=delay
  Delay21 : xbsIndex_r4/Delay  rst=off  infoeditControl=Selection of Reset will increase slice count due to use of real FFs and instead of SRLs  en=off  latency=8  reg_retiming=off  dbl_ovrd=off  block_type=delay
  Delay22 : xbsIndex_r4/Delay  rst=off  infoeditControl=Selection of Reset will increase slice count due to use of real FFs and instead of SRLs  en=off  latency=7  reg_retiming=off  dbl_ovrd=off  block_type=delay
  Delay23 : xbsIndex_r4/Delay  rst=off  infoeditControl=Selection of Reset will increase slice count due to use of real FFs and instead of SRLs  en=off  latency=2  reg_retiming=off  dbl_ovrd=off  block_type=delay
  Delay24 : xbsIndex_r4/Delay  rst=off  infoeditControl=Selection of Reset will increase slice count due to use of real FFs and instead of SRLs  en=off  latency=4  reg_retiming=off  dbl_ovrd=off  block_type=delay
  Delay6 : xbsIndex_r4/Delay  rst=off  infoeditControl=Selection of Reset will increase slice count due to use of real FFs and instead of SRLs  en=off  latency=3  reg_retiming=off  dbl_ovrd=off  block_type=delay
  Delay7 : xbsIndex_r4/Delay  rst=off  infoeditControl=Selection of Reset will increase slice count due to use of real FFs and instead of SRLs  en=off  latency=3  reg_retiming=off  dbl_ovrd=off  block_type=delay
  Delay8 : xbsIndex_r4/Delay  rst=off  infoeditControl=Selection of Reset will increase slice count due to use of real FFs and instead of SRLs  en=off  latency=4  reg_retiming=off  dbl_ovrd=off  block_type=delay
  Relational{,1..11} (12 alike) : xbsIndex_r4/Relational  mode=a>b  op_type=Bool  en=off  latency=1  dbl_ovrd=off  block_type=relational
  Shift{,1..3} (4 alike) : xbsIndex_r4/Shift  shift_dir=Right  shift_bits=1  en=off  latency=1  precision=Full  arith_type="Signed  (2's comp)"  n_bits=16  bin_pt=14  quantization=Truncate  overflow=Wrap  dbl_ovrd=off  block_type=shift
  Out1 : Outport
  wires:
  Convert/1 -> Delay14/1
  Convert11/1 -> AddSub20/2
  Convert10/1 -> AddSub14/2
  Convert9/1 -> AddSub24/2
  Convert8/1 -> AddSub18/2
  Convert7/1 -> AddSub23/2
  Convert6/1 -> AddSub22/2
  Convert5/1 -> AddSub21/2
  Convert4/1 -> AddSub19/2
  Convert3/1 -> AddSub17/2
  Convert2/1 -> AddSub15/2
  Convert1/1 -> AddSub16/2
  Delay14/1 -> AddSub16/1
  Delay25/1 -> Relational11/1
  Delay13/1 -> Delay25/1, Relational10/1
  Delay12/1 -> Delay13/1, Relational9/1
  Delay11/1 -> Relational8/1, Delay12/1
  Delay10/1 -> Relational7/1, Delay11/1
  Delay9/1 -> AddSub21/1
  Delay8/1 -> Relational6/1, Delay10/1
  Delay7/1 -> AddSub5/1, AddSub5/2
  Delay6/1 -> AddSub6/2
  Delay5/1 -> Relational5/1
  Delay4/1 -> Relational4/1
  Delay3/1 -> Delay4/1, Delay8/1, Relational3/1
  Delay2/1 -> Delay15/1, Relational1/1
  Delay1/1 -> Relational/1, Delay2/1
  d2_ticks/1 -> Shift1/1
  d4_ticks/1 -> Shift3/1
  AddSub14/1 -> Out1/1
  Relational9/1 -> Convert8/1
  Relational7/1 -> Convert6/1
  Shift3/1 -> Delay21/1
  AddSub21/1 -> AddSub22/1
  AddSub2/1 -> Relational3/2, AddSub3/1
  Relational11/1 -> Convert10/1
  Relational3/1 -> Convert3/1
  Shift2/1 -> Delay20/1
  d0_ticks/1 -> CMult/1
  Delay24/1 -> AddSub13/2
  AddSub13/1 -> Relational11/2
  d1_ticks/1 -> Shift/1
  AddSub10/1 -> Relational8/2, AddSub11/1
  AddSub3/1 -> Delay5/1, Relational4/2, AddSub4/1
  AddSub22/1 -> AddSub23/1
  AddSub1/1 -> Relational2/2, AddSub2/1
  Relational/1 -> Convert/1
  AddSub17/1 -> AddSub19/1
  Delay18/1 -> AddSub3/2
  AddSub19/1 -> AddSub20/1
  Relational10/1 -> Convert9/1
  Relational6/1 -> Convert5/1
  d3_ticks/1 -> Shift2/1
  Delay21/1 -> AddSub10/2, Delay23/1
  Relational2/1 -> Convert2/1
  AddSub7/1 -> AddSub8/1, Relational6/2
  Delay15/1 -> Relational2/1, Delay3/1
  AddSub8/1 -> Relational7/2, AddSub10/1
  AddSub/1 -> Relational1/2, AddSub1/1
  AddSub4/1 -> Relational5/2, AddSub6/1
  Relational5/1 -> Convert11/1
  Delay23/1 -> AddSub12/2
  AddSub23/1 -> AddSub18/1
  Relational8/1 -> Convert7/1
  AddSub12/1 -> Relational10/2, AddSub13/1
  Relational1/1 -> Convert1/1
  Delay16/1 -> AddSub1/2, Delay18/1
  AddSub5/1 -> AddSub7/2
  Delay22/1 -> AddSub11/2
  Delay20/1 -> AddSub8/2, Delay24/1
  Shift/1 -> AddSub/2, Delay19/1
  CMult/1 -> Relational/2, AddSub/1, Delay17/1
  AddSub18/1 -> AddSub24/1
  counter/1 -> Delay1/1
  Delay19/1 -> AddSub4/2
  Relational4/1 -> Convert4/1
  AddSub6/1 -> AddSub7/1
  AddSub11/1 -> Relational9/2, AddSub12/1
  AddSub20/1 -> Delay9/1
  Delay17/1 -> Delay6/1, Delay7/1, Delay22/1, AddSub2/2
  Shift1/1 -> Delay16/1
  AddSub24/1 -> AddSub14/1
  AddSub16/1 -> AddSub15/1
  AddSub15/1 -> AddSub17/1
